simulink library "commdigpbndfm2"  (Simulink 5.0)
undefined symbols (not defined in the file or in its folder): D
libraries: commblksprivate x4, dspsigattribs x2, commdigbbndfm2 x2, dspsigops x1
settings Model: RequirementInfo=9  CovMetricSettings=d  Creator=tdelve  LastModifiedBy=mmclerno

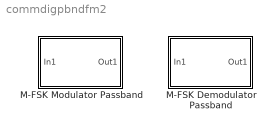
== system commdigpbndfm2 ==
  M-FSK Demodulator Passband : Subsystem  mask(M-FSK Demodulator Passband){M=8, OutType=Integer, Dec=Binary, freqSep=100, td=1/100, numSamp=10, Fc=3000, Ph=0, InSamp=1/10000}
      mask prompts: M "M-ary number:"; OutType "Output type:"; Dec "Symbol set ordering:"; freqSep "Frequency separation (Hz):"; td "Symbol period (s):"; numSamp "Baseband samples per symbol:"; Fc "Carrier frequency (Hz):"; Ph "Carrier initial phase (rad):"; InSamp "Input sample time (s):"
      mask help:
      | Demodulate the input signal using the frequency shift keying method.
      |
      | The input signal must be a sample-based scalar. In case of bit output, the width of the output is the number of bits per symbol. The symbols can be either binary-demapped or Gray-demapped into bits.
      |
      | The symbol period divided by the baseband samples per symbol must be an integer multiple of the input sample time.
      mask init:
      | commblkdyampmdemod('M-FSK Demodulator Baseband','update');
      | commblkpbndfskdemod(gcb,'init');
      settings: RTWFcnNameOpts=Auto  RTWFileNameOpts=Auto
      mask Help: helpview(commbhelp)
      mask StyleString: edit,popup(Bit|Integer),popup(Binary|Gray),edit,edit,edit,edit,edit,edit
      mask CallbackString: |commblkpbndfskdemod(gcb,'InType');|||||||
      mask Display:
      | plot(0,0,100,100,[5+1.5*[[0:.8:10] [10:1.6:20] [20:.8:30]] 50 50 50 50+15*[0 1 1 2 2 3]],[85+10*[sin([0:.8:10]*pi*2/5) sin([10:1.6:20]*pi/5) sin([20:.8:30]*pi*2/5)] 85 99 75 85+8*[1 1 -1 -1 1 1]]);
      | text(51,51,'M-FSK','horiz','center','verti','middle');
  M-FSK Modulator Passband : Subsystem  mask(M-FSK Modulator Passband){M=8, InType=Integer, Enc=Binary, freqSep=100, phaseType=Continuous, td=1/100, numSamp=10, Fc=3000, Ph=0, OutSamp=1/10000}
      mask prompts: M "M-ary number:"; InType "Input type:"; Enc "Symbol set ordering:"; freqSep "Frequency separation (Hz):"; phaseType "Phase continuity:"; td "Symbol period (s):"; numSamp "Baseband samples per symbol:"; Fc "Carrier frequency (Hz):"; Ph "Carrier initial phase (rad):"; OutSamp "Output sample time (s):"
      mask help:
      | Modulate the input signal using the frequency shift keying method.
      |
      | The input signal must be sample-based. In case of integer input, the input must be a scalar. In case of bit input, the width of the input must equal the number of bits per symbol. The bits can be either binary-mapped or Gray-mapped into symbols.
      |
      | The input sample time must equal the symbol period.  Also, the symbol period divided by the baseband samples per symbol must be an integer multiple of the output sample time.
      mask init:
      | commblkdyampmmod('M-FSK Modulator Baseband','update');
      | commblkpbndfskmod(gcb,'init');
      settings: RTWFcnNameOpts=Auto  RTWFileNameOpts=Auto
      mask Help: helpview(commbhelp)
      mask StyleString: edit,popup(Bit|Integer),popup(Binary|Gray),edit,popup(Continuous|Discontinuous),edit,edit,edit,edit,edit
      mask CallbackString: |commblkpbndfskmod(gcb,'InType');||||||||
      mask Display:
      | plot(0,0,100,100,[5+15*[0 1 1 2 2 3] 50 50 50 50+1.5*[[0:.8:10] [10:1.6:20] [20:.8:30]]],[85+8*[1 1 -1 -1 1 1] 85 99 75 85+10*[sin([0:.8:10]*pi*2/5) sin([10:1.6:20]*pi/5) sin([20:.8:30]*pi*2/5)]]);
      | disp('M-FSK')

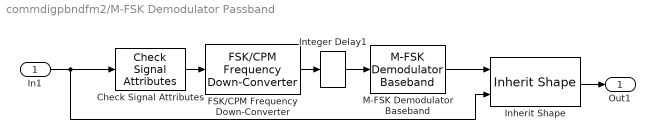
== system commdigpbndfm2/M-FSK Demodulator Passband ==
  In1 : Inport  Port=1  LatchInput=off
  Check Signal Attributes : dspsigattribs/Check Signal Attributes  SigAttribCheckMethod=Matches attributes exactly  Complexity=Ignore  Frame=Frame-based  DimsCheckMethod=Ignore  Dimensions=1-D  DatatypeCheckMethod=Ignore  DatatypeGeneral=Boolean  DtypeFloatSpecific=Any floating-point  DtypeFixedSpecific=Any fixed-point  DtypeIntSpecific=Any integer  SampleMode=Ignore
  FSK/CPM Frequency Down-Converter : commblksprivate/FSK//CPM Frequency Down-Converter  AncestorBlock=|  modType=FSK  M=M  freqSep=freqSep  td=td  Fc=Fc  Ph=Ph  Tin=InSamp  Tout=td / numSamp
      | commblksprivate/FSK//CPM
      | Frequency
      | Down-Converter
  Inherit Shape : commblksprivate/Inherit Shape
  Integer Delay1 : dspsigops/Integer Delay  delay=numSamp-1  ic=0
  M-FSK Demodulator Baseband : commdigbbndfm2/M-FSK Demodulator Baseband  M=M  OutType=Integer  Dec=Binary  freqSep=freqSep  numSamp=numSamp
  Out1 : Outport  Port=1
  wires:
  Check Signal Attributes/1 -> FSK/CPM Frequency Down-Converter/1
  M-FSK Demodulator Baseband/1 -> Inherit Shape/1
  FSK/CPM Frequency Down-Converter/1 -> Integer Delay1/1
  Integer Delay1/1 -> M-FSK Demodulator Baseband/1
  In1/1 -> Check Signal Attributes/1, Inherit Shape/2
  Inherit Shape/1 -> Out1/1

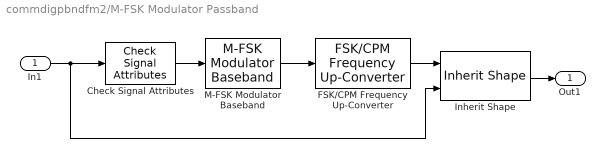
== system commdigpbndfm2/M-FSK Modulator Passband ==
  In1 : Inport  Port=1  LatchInput=off
  Check Signal Attributes : dspsigattribs/Check Signal Attributes  SigAttribCheckMethod=Matches attributes exactly  Complexity=Ignore  Frame=Frame-based  DimsCheckMethod=Ignore  Dimensions=1-D  DatatypeCheckMethod=Ignore  DatatypeGeneral=Boolean  DtypeFloatSpecific=Any floating-point  DtypeFixedSpecific=Any fixed-point  DtypeIntSpecific=Any integer  SampleMode=Ignore
  FSK/CPM Frequency Up-Converter : commblksprivate/FSK//CPM Frequency Up-Converter  modType=FSK  M=M  freqSep=freqSep  td=td  Fc=Fc  Ph=Ph  Tin=td / numSamp  Tout=OutSamp
  Inherit Shape : commblksprivate/Inherit Shape
  M-FSK Modulator Baseband : commdigbbndfm2/M-FSK Modulator Baseband  M=M  InType=Integer  Enc=Binary  freqSep=freqSep  phaseType=Continuous  numSamp=numSamp
  Out1 : Outport  Port=1
  wires:
  M-FSK Modulator Baseband/1 -> FSK/CPM Frequency Up-Converter/1
  FSK/CPM Frequency Up-Converter/1 -> Inherit Shape/1
  Check Signal Attributes/1 -> M-FSK Modulator Baseband/1
  In1/1 -> Check Signal Attributes/1, Inherit Shape/2
  Inherit Shape/1 -> Out1/1
